simulink model "hacheur_serie_2"  (R2018a)
settings: Solver=ode15s  StartTime=0.0  StopTime=0.1  RelTol=1e-3  EnableMultiTasking=on
libraries: fl_lib x8, nesl_utility x6, elec_lib x1, pe_lib x1
settings Model: Creator=Ivan  LastModifiedBy=Ivan
settings DataIOCC: LimitDataPoints=on  SaveFormat=Array  SignalLoggingSaveFormat=ModelDataLogs
settings OptimizationCC: LifeSpan=inf
settings DebuggingCC: UnderspecifiedInitializationDetection=Classic  MergeDetectMultiDrivingBlocksExec=none  SolverPrmCheckMsg=warning  MultiTaskDSMMsg=warning  MultiTaskCondExecSysMsg=none  AllowSymbolicDim=off  StateNameClashWarn=warning  SFUnexpectedBacktrackingDiag=warning  SFNoUnconditionalDefaultTransitionDiag=warning  SFExecutionAtInitializationDiag=none
settings HardwareCC: ProdBitPerPointer=32  ProdBitPerSizeT=32  ProdBitPerPtrDiffT=32  ProdLargestAtomicFloat=None  ProdIntDivRoundTo=Undefined  ProdEndianess=Unspecified  ProdWordSize=32  ProdHWDeviceType=32-bit Generic
settings ModelReferenceCC: PropagateSignalLabelsOutOfModel=off
settings CodeAppCC: StateflowObjectComments=on
settings GRTTargetCC: TargetLangStandard=C89/C90 (ANSI)  GeneratePreprocessorConditionals=Disable all
settings ConfigComp: CovMetricSettings=dw  CovHtmlReporting=on  CovSaveCumulativeToWorkspaceVar=on  CovSaveSingleToWorkspaceVar=on  CovExternalEMLEnable=off
settings SimscapeCC: SimscapeNormalizeSystem=off

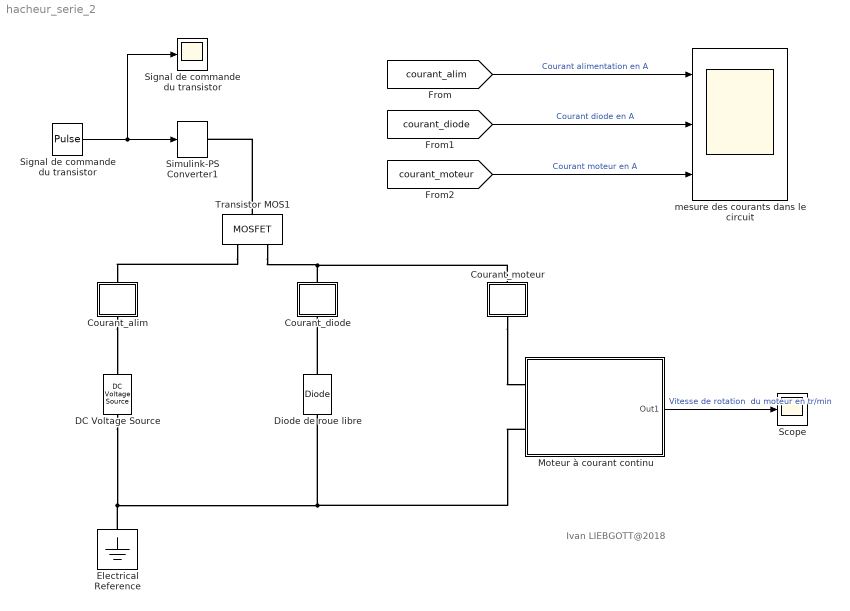
== system hacheur_serie_2 ==
  note: Ivan LIEBGOTT@2018
  " Signal de commande du transistor" : DiscretePulseGenerator  PulseType=Time based  Period=0.1  PulseWidth=50
  Courant_alim : Subsystem
  Courant_diode : Subsystem
  Courant_moteur : Subsystem
  DC Voltage Source : fl_lib/Electrical/Electrical Sources/DC Voltage Source  v0=24 V
  Diode de roue libre : fl_lib/Electrical/Electrical Elements/Diode  Vf=0.1 V  Ron=0.1 Ohm  Goff=1e-8 1/Ohm  i_specify=off  i_priority=High  i=0 A  i_nominal_specify=off  i_nominal_unit=A  i_nominal_value=1  v_specify=off  v_priority=High  v=0 V  v_nominal_specify=off  v_nominal_unit=V  v_nominal_value=1
  Electrical Reference : fl_lib/Electrical/Electrical Elements/Electrical Reference
  Moteur à courant continu : Subsystem
      mask Display: image('moteur_CC.jpg')
  Scope : Scope
  Signal de commande du transistor : Scope
  Simulink-PS Converter1 : nesl_utility/Simulink-PS Converter  PhysicalDomain=network_engine_domain  SubClassName=ps_input  LeftPortType=input  RightPortType=output  PseudoPeriodic=off  Frequencies=[]  NoiseDistribution=none  NoiseParameters=[]  Unit=1  AffineConversion=off  FilteringAndDerivatives=zero  SimscapeFilterOrder=1  InputFilterTimeConstant=0.001  UdotUserProvided=1
  Transistor MOS1 : pe_lib/Semiconductors/Fundamental Components/MOSFET  Rds=0.01 Ohm  Goff=1e-6 1/Ohm  Vth=0.5 V  diode_param=1  diode_Vf=0.8 V  diode_Ron=0.001 Ohm  diode_Goff=1e-5 1/Ohm  diode_C=5e-8 F  diode_iRM=-235 A  diode_iF=300 A  diode_idot=-50 A/us  diode_trr_param=1  diode_trr_factor=3  diode_trr=15 us  diode_Qrr=1.5e+3 s*uA  thermal_loss_option=2  Voff=300 V  Tau=1e-4 s  Tj=[ 298.15 398.15 ] K  Iout_scalar=600 A  Eon_scalar=0.02286 J  Eoff_scalar=0.01714 J  Von_scalar=2.7 V  Iout_data=[ 0 10 50 100 200 400 600 ] A  Eon_data=[ 0 2.9e-4 0.00143 0.00286 0.00571 0.01314 0.02286; 0 5.7e-4 0.00263 0.00514 0.01029 0.02057 0.03029 ] J  Eoff_data=[ 0 2.1e-4 0.00107 0.00214 0.00429 0.009859999999999999 0.01714; 0 4.3e-4 0.00197 0.00386 0.00771 0.01543 0.02271 ] J  Von_data=[ 0 1.1 1.3 1.45 1.75 2.25 2.7; 0 1 1.15 1.35 1.7 2.35 3 ] V
      settings: SourceProductName=Simscape Power Systems  SourceProductBaseCode=PS
  mesure des courants dans le circuit : Scope  NumInputPorts=3
  wires:
  " Signal de commande du transistor"/1 -> Signal de commande du transistor/1, Simulink-PS Converter1/1
  Moteur à courant continu/1(Out1) -> Scope/1  "Vitesse de rotation  du moteur en tr/min"
  [courant_alim] -> mesure des courants dans le circuit/1  "Courant alimentation en A"
  [courant_diode] -> mesure des courants dans le circuit/2  "Courant diode en A"
  [courant_moteur] -> mesure des courants dans le circuit/3  "Courant moteur en A"
  connections:
  Transistor MOS1/LConn1 -- Simulink-PS Converter1/RConn1
  DC Voltage Source/RConn1 -- Electrical Reference/LConn1 -- Moteur à courant continu/LConn2 -- Diode de roue libre/LConn1
  Courant_diode/RConn1 -- Transistor MOS1/RConn2 -- Courant_moteur/LConn1
  Transistor MOS1/RConn1 -- Courant_alim/RConn1
  Courant_alim/LConn1 -- DC Voltage Source/LConn1
  Diode de roue libre/RConn1 -- Courant_diode/LConn1
  Courant_moteur/RConn1 -- Moteur à courant continu/LConn1

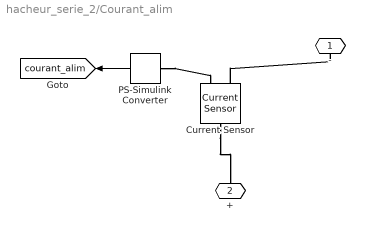
== system hacheur_serie_2/Courant_alim ==
  Current Sensor : fl_lib/Electrical/Electrical Sensors/Current Sensor
  PS-Simulink Converter : nesl_utility/PS-Simulink Converter  PhysicalDomain=network_engine_domain  SubClassName=ps_output  LeftPortType=input  RightPortType=output  PseudoPeriodic=off  Frequencies=[]  Unit=1  AffineConversion=off
  - : PMIOPort  Side=Right
  + : PMIOPort  Port=2  Side=Left
  tag scope: courant_alim=global
  wires:
  PS-Simulink Converter/1 -> [courant_alim]
  connections:
  Current Sensor/LConn1 -- +/RConn1
  PS-Simulink Converter/LConn1 -- Current Sensor/RConn1
  Current Sensor/RConn2 -- -/RConn1

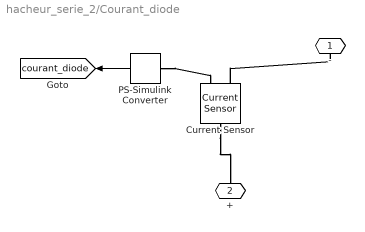
== system hacheur_serie_2/Courant_diode ==
  Current Sensor : fl_lib/Electrical/Electrical Sensors/Current Sensor
  PS-Simulink Converter : nesl_utility/PS-Simulink Converter  PhysicalDomain=network_engine_domain  SubClassName=ps_output  LeftPortType=input  RightPortType=output  PseudoPeriodic=off  Frequencies=[]  Unit=1  AffineConversion=off
  - : PMIOPort  Side=Right
  + : PMIOPort  Port=2  Side=Left
  tag scope: courant_diode=global
  wires:
  PS-Simulink Converter/1 -> [courant_diode]
  connections:
  Current Sensor/RConn2 -- -/RConn1
  PS-Simulink Converter/LConn1 -- Current Sensor/RConn1
  Current Sensor/LConn1 -- +/RConn1

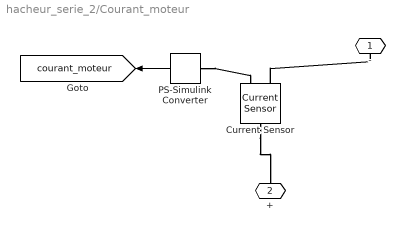
== system hacheur_serie_2/Courant_moteur ==
  Current Sensor : fl_lib/Electrical/Electrical Sensors/Current Sensor
  PS-Simulink Converter : nesl_utility/PS-Simulink Converter  PhysicalDomain=network_engine_domain  SubClassName=ps_output  LeftPortType=input  RightPortType=output  PseudoPeriodic=off  Frequencies=[]  Unit=1  AffineConversion=off
  - : PMIOPort  Side=Right
  + : PMIOPort  Port=2  Side=Left
  tag scope: courant_moteur=global
  wires:
  PS-Simulink Converter/1 -> [courant_moteur]
  connections:
  Current Sensor/LConn1 -- +/RConn1
  PS-Simulink Converter/LConn1 -- Current Sensor/RConn1
  Current Sensor/RConn2 -- -/RConn1

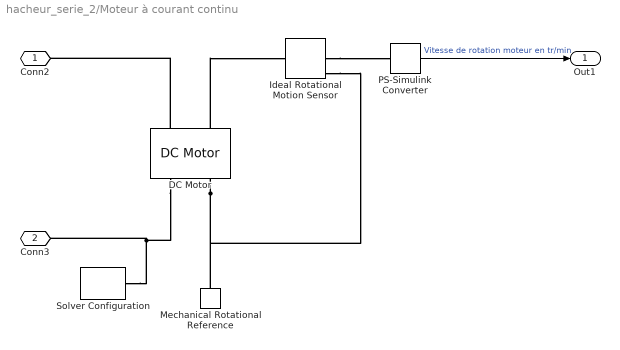
== system hacheur_serie_2/Moteur à courant continu ==
  DC Motor : elec_lib/Actuators & Drivers/Rotational Actuators/DC Motor  parameterization=1  Ra=20 Ohm  La=100 mH  emf_or_torque=1  Kv=9e-4 V/rpm  Ki=6.876e-4 N*m/A  T_stall=2.4e-4 N*m  w_max=1.91e+4 rpm  w_rated=1.5e+4 rpm  P_rated=0.08 W  V_rated=1.5 V  J=0.5 g*cm^2  lam_param=1  lam=0.001 N*m/(rad/s)  i_noload=0 A  V_i_noload=1.5 V  speed0=0 rpm  alpha=0.00393 1/K  Tmeas=25 C  thermal_mass=100 J/K  initial_temperature=25 C
  Ideal Rotational Motion Sensor : fl_lib/Mechanical/Mechanical Sensors/Ideal Rotational Motion Sensor  offset=0 rad
  Mechanical Rotational Reference : fl_lib/Mechanical/Rotational Elements/Mechanical Rotational Reference
  PS-Simulink Converter : nesl_utility/PS-Simulink Converter  PhysicalDomain=network_engine_domain  SubClassName=ps_output  LeftPortType=input  RightPortType=output  PseudoPeriodic=off  Frequencies=[]  Unit=rpm  AffineConversion=off
  Solver Configuration : nesl_utility/Solver Configuration  PhysicalDomain=network_engine_domain  SubClassName=solver  LeftPortType=input  RightPortType=generic  Tones=[]  Harmonics=[]  SimulateNoise=off  Profile=off  UseLocalSampling=off  EnableSwitchedLinearOptims=on  FrequencyDomain=off  UseCCode=off  RelTol=0.001  AbsTol=1e-06  MinStep=1e-09  ToWorkspace=off  RevertToSquareIcSolve=off  NumHomotopyIterations=100  PhasorMode=off  PhasorModeNumHarmonics=1  DoDC=off  ResidualTolerance=1e-09  UseLocalSolver=off  LocalSolverChoice=NE_BACKWARD_EULER_ADVANCER  LocalSolverSampleTime=0.001  DoFixedCost=off  MaxNonlinIter=3  MaxModeIter=2  LinearAlgebra=Sparse  EquationFormulation=NE_TIME_EF  DelaysMemoryBudget=1024  AutomaticFiltering=on  FilteringTimeConstant=0.001
  Conn2 : PMIOPort  Side=Left
  Conn3 : PMIOPort  Port=2  Side=Left
  Out1 : Outport
  wires:
  PS-Simulink Converter/1 -> Out1/1  "Vitesse de rotation moteur en tr/min"
  connections:
  DC Motor/RConn1 -- Solver Configuration/RConn1 -- Conn3/RConn1
  DC Motor/LConn2 -- Ideal Rotational Motion Sensor/LConn1
  Ideal Rotational Motion Sensor/RConn2 -- PS-Simulink Converter/LConn1
  DC Motor/RConn2 -- Ideal Rotational Motion Sensor/RConn1 -- Mechanical Rotational Reference/LConn1
  DC Motor/LConn1 -- Conn2/RConn1
